simulink model "SistemaP2"  (R2023a)
settings: Solver=VariableStepAuto  StartTime=0.0  StopTime=30.0  RelTol=1e-3
libraries: slpidlib x1
settings Model: LastModifiedBy=andre
settings DataIOCC: ReturnWorkspaceOutputs=off  TimeSaveName=t
settings DebuggingCC: AlgebraicLoopMsg=none  ArtificialAlgebraicLoopMsg=none
settings RTWCC: GPUComputeCapability=5.0

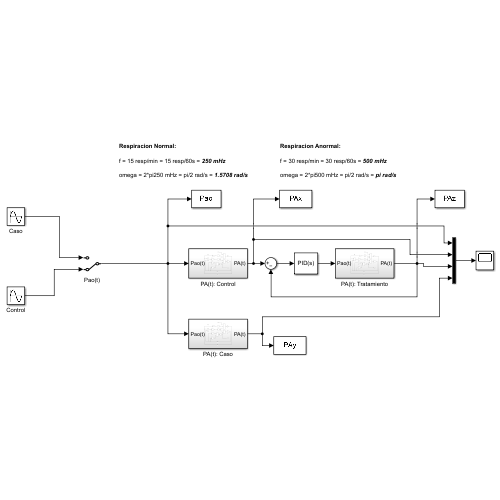
[thumbnail: Simulink's stored preview of the top-level diagram]
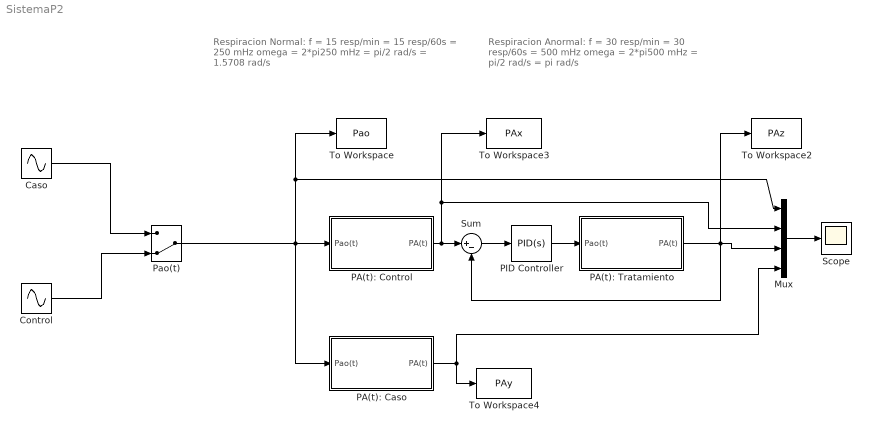
== system SistemaP2 ==
  note: Respiracion Anormal:
      |
      | f = 30 resp/min = 30 resp/60s = 500 mHz
      |
      | omega = 2*pi500 mHz = pi/2 rad/s = pi rad/s
  note: Respiracion Normal:
      |
      | f = 15 resp/min = 15 resp/60s = 250 mHz
      |
      | omega = 2*pi250 mHz = pi/2 rad/s = 1.5708 rad/s
  Caso : Sin  Amplitude=1.5  Frequency=pi  SampleTime=0
  Control : Sin  Amplitude=2.5  Frequency=1.5708  SampleTime=0
  Mux : Mux
  PA(t): Caso : Subsystem
  PA(t): Control : Subsystem
  PA(t): Tratamiento : Subsystem
  PID Controller : slpidlib/PID Controller  Controller=PID  Form=Parallel  TimeDomain=Continuous-time  UseExternalTs=off  SampleTime=-1  IntegratorMethod=Forward Euler  FilterMethod=Forward Euler  ControllerParametersSource=internal  P=173.172262760122  I=4050.38640713002  UseKiTs=off  D=0.822077023906802  N=16708.0113456375  UseFilter=on  TunerSelectOption=Transfer Function Based (PID Tuner App)  InitialConditionSource=internal  InitialConditionForIntegrator=0  InitialConditionForFilter=0  DifferentiatorICPrevScaledInput=0  ExternalReset=none  TrackingMode=off  Kt=1  LimitOutput=off  SatLimitsSource=internal  UpperSaturationLimit=inf  LowerSaturationLimit=-inf  LinearizeAsGain=on  AntiWindupMode=none  Kb=1  LimitIntegrator=off  UpperIntegratorSaturationLimit=inf  LowerIntegratorSaturationLimit=-inf  POutMin=[]  POutMax=[]  IOutMin=[]  IOutMax=[]  DOutMin=[]  DOutMax=[]  NOutMin=[]  NOutMax=[]  SumOutMin=[]  SumOutMax=[]  SaturationOutMin=[]  SaturationOutMax=[]  PParamMin=[]  PParamMax=[]  IParamMin=[]  IParamMax=[]  DParamMin=[]  DParamMax=[]  NParamMin=[]  NParamMax=[]  KbParamMin=[]  KbParamMax=[]  KtParamMin=[]  KtParamMax=[]  KbOutMin=[]  KbOutMax=[]  KtOutMin=[]  KtOutMax=[]  IntegratorOutMin=[]  IntegratorOutMax=[]  FilterOutMin=[]  FilterOutMax=[]  SumI1OutMin=[]  SumI1OutMax=[]  SumI2OutMin=[]  SumI2OutMax=[]  SumI3OutMin=[]  SumI3OutMax=[]  SumI4OutMin=[]  SumI4OutMax=[]  SumDOutMin=[]  SumDOutMax=[]  DifferentiatorOutMin=[]  DifferentiatorOutMax=[]  FilterDiffOutCoefMin=[]  FilterDiffOutCoefMax=[]  ReciprocalOutMin=[]  ReciprocalOutMax=[]  SumDenOutMin=[]  SumDenOutMax=[]  SumNumOutMin=[]  SumNumOutMax=[]  DivideOutMin=[]  DivideOutMax=[]  UdiffTsProdOutMin=[]  UdiffTsProdOutMax=[]  NTsProdOutMin=[]  NTsProdOutMax=[]  UintegralTsProdOutMin=[]  UintegralTsProdOutMax=[]  UngainTsProdOutMin=[]  UngainTsProdOutMax=[]  ClampingZeroOutDataTypeStr=Inherit: Inherit via back propagation  ClampingZeroOutMin=[]  ClampingZeroOutMax=[]  FilterDenConstantOutDataTypeStr=Inherit: Inherit via back propagation  FilterDenConstantOutMin=[]  FilterDenConstantOutMax=[]  PCopyOutDataTypeStr=Inherit: Inherit via back propagation  PCopyOutMin=[]  PCopyOutMax=[]  NCopyOutDataTypeStr=Inherit: Inherit via back propagation  NCopyOutMin=[]  NCopyOutMax=[]  IntegratorContinuousStateAttributes=''  IntegratorStateMustResolveToSignalObject=off  IntegratorRTWStateStorageClass=Auto  FilterContinuousStateAttributes=''  FilterStateMustResolveToSignalObject=off  FilterRTWStateStorageClass=Auto  ParallelPVariant=InternalParameters  IdealPVariant=Disabled  IVariant=InternalParameters  DVariant=InternalParameters  IntegratorVariant=Continuous  SatVariant=Disabled  AWVariant=Passthrough  PCopyVariant=Disabled  TRVariant=Disabled  FdbkBlocksVariant=Forward  IdealPFdbkVariant=Disabled  SatFdbkVariant=Disabled  DerivativeFilterVariant=ContFilter  NVariant=InternalParameters  NCopyVariant=Disabled  FilterICVariant=InternalICsFilter  IntegratorICVariant=InternalICs  ExternalResetVariant=Disabled  TRSumVariant=Passthrough  SumFdbkVariant=Disabled  SumVariant=Sum_PID  TsampFilterVariant=InternalTs  TsampNgainVariant=Passthrough  TsampIntegralVariant=Disabled_SignalSpec  ExternalSaturationOutDataTypeStr=Inherit: Same as second input
  Pao(t) : ManualSwitch  CurrentSetting=0
  Scope : Scope
  Sum : Sum  Inputs=|+-
  To Workspace : ToWorkspace  VariableName=Pao  SampleTime=-1
  To Workspace2 : ToWorkspace  VariableName=PAz  SampleTime=-1
  To Workspace3 : ToWorkspace  VariableName=PAx  SampleTime=-1
  To Workspace4 : ToWorkspace  VariableName=PAy  SampleTime=-1
  wires:
  Mux/1 -> Scope/1
  Sum/1 -> PID Controller/1
  PID Controller/1 -> PA(t): Tratamiento/1(Pao(t))
  PA(t): Caso/1(PA(t)) -> Mux/4, To Workspace4/1
  PA(t): Control/1(PA(t)) -> Sum/1, Mux/2, To Workspace3/1
  PA(t): Tratamiento/1(PA(t)) -> Sum/2, To Workspace2/1, Mux/3
  Caso/1 -> Pao(t)/1
  Pao(t)/1 -> PA(t): Caso/1(Pao(t)), To Workspace/1, Mux/1, PA(t): Control/1(Pao(t))
  Control/1 -> Pao(t)/2

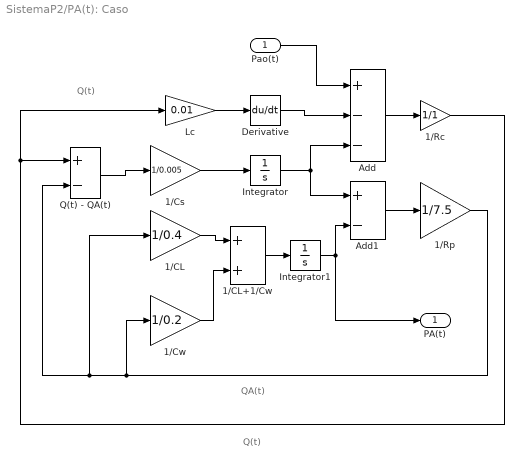
== system SistemaP2/PA(t): Caso ==
  note: QA(t)
  note: Q(t)
  note: Q(t)
  Pao(t) : Inport
  1/CL : Gain  Gain=1/0.4
  1/CL+1/Cw : Sum
  1/Cs : Gain  Gain=1/0.005
  1/Cw : Gain  Gain=1/0.2
  1/Rc : Gain  Gain=1/1
  1/Rp : Gain  Gain=1/7.5
  Add : Sum  Inputs=+--
  Add1 : Sum  Inputs=+-
  Derivative : Derivative
  Integrator : Integrator
  Integrator1 : Integrator
  Lc : Gain  Gain=0.01
  Q(t) - QA(t) : Sum  Inputs=+-
  PA(t) : Outport
  wires:
  1/Cw/1 -> 1/CL+1/Cw/2
  1/Rc/1 -> Lc/1, Q(t) - QA(t)/1
  1/CL/1 -> 1/CL+1/Cw/1
  Add1/1 -> 1/Rp/1
  1/CL+1/Cw/1 -> Integrator1/1
  1/Rp/1 -> 1/CL/1, Q(t) - QA(t)/2, 1/Cw/1
  Integrator1/1 -> PA(t)/1, Add1/2
  Lc/1 -> Derivative/1
  Derivative/1 -> Add/2
  1/Cs/1 -> Integrator/1
  Q(t) - QA(t)/1 -> 1/Cs/1
  Integrator/1 -> Add1/1, Add/3
  Pao(t)/1 -> Add/1
  Add/1 -> 1/Rc/1

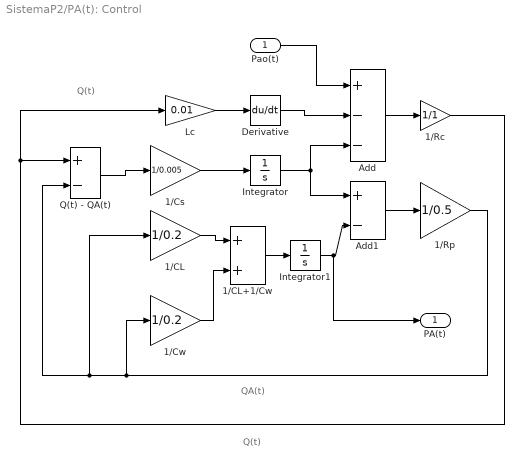
== system SistemaP2/PA(t): Control ==
  note: QA(t)
  note: Q(t)
  note: Q(t)
  Pao(t) : Inport
  1/CL : Gain  Gain=1/0.2
  1/CL+1/Cw : Sum
  1/Cs : Gain  Gain=1/0.005
  1/Cw : Gain  Gain=1/0.2
  1/Rc : Gain  Gain=1/1
  1/Rp : Gain  Gain=1/0.5
  Add : Sum  Inputs=+--
  Add1 : Sum  Inputs=+-
  Derivative : Derivative
  Integrator : Integrator
  Integrator1 : Integrator
  Lc : Gain  Gain=0.01
  Q(t) - QA(t) : Sum  Inputs=+-
  PA(t) : Outport
  wires:
  1/Cw/1 -> 1/CL+1/Cw/2
  1/Rc/1 -> Lc/1, Q(t) - QA(t)/1
  1/CL/1 -> 1/CL+1/Cw/1
  Add1/1 -> 1/Rp/1
  1/CL+1/Cw/1 -> Integrator1/1
  1/Rp/1 -> 1/CL/1, Q(t) - QA(t)/2, 1/Cw/1
  Integrator1/1 -> PA(t)/1, Add1/2
  Lc/1 -> Derivative/1
  Derivative/1 -> Add/2
  1/Cs/1 -> Integrator/1
  Q(t) - QA(t)/1 -> 1/Cs/1
  Integrator/1 -> Add1/1, Add/3
  Pao(t)/1 -> Add/1
  Add/1 -> 1/Rc/1

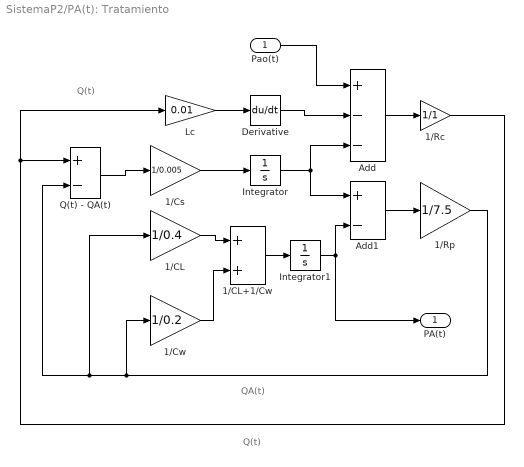
== system SistemaP2/PA(t): Tratamiento ==
  note: Q(t)
  note: Q(t)
  note: QA(t)
  Pao(t) : Inport
  1/CL : Gain  Gain=1/0.4
  1/CL+1/Cw : Sum
  1/Cs : Gain  Gain=1/0.005
  1/Cw : Gain  Gain=1/0.2
  1/Rc : Gain  Gain=1/1
  1/Rp : Gain  Gain=1/7.5
  Add : Sum  Inputs=+--
  Add1 : Sum  Inputs=+-
  Derivative : Derivative
  Integrator : Integrator
  Integrator1 : Integrator
  Lc : Gain  Gain=0.01
  Q(t) - QA(t) : Sum  Inputs=+-
  PA(t) : Outport
  wires:
  Pao(t)/1 -> Add/1
  Derivative/1 -> Add/2
  Lc/1 -> Derivative/1
  Integrator/1 -> Add1/1, Add/3
  Add/1 -> 1/Rc/1
  1/Rc/1 -> Lc/1, Q(t) - QA(t)/1
  1/Cs/1 -> Integrator/1
  Q(t) - QA(t)/1 -> 1/Cs/1
  Add1/1 -> 1/Rp/1
  1/Rp/1 -> 1/CL/1, Q(t) - QA(t)/2, 1/Cw/1
  1/Cw/1 -> 1/CL+1/Cw/2
  1/CL+1/Cw/1 -> Integrator1/1
  Integrator1/1 -> Add1/2, PA(t)/1
  1/CL/1 -> 1/CL+1/Cw/1
